simulink model "s_c_nbe_m1k_dbg2"  (R2016b)
(part 3 of 55)

  phase0/2(in_delta) -> Reinterpret3/1
  Reinterpret8/1 -> Concat22/1
  Reinterpret1/1 -> Concat22/2
  Reinterpret2/1 -> Concat22/3
  Reinterpret3/1 -> Concat22/4
  phase1/1(in_initial) -> Reinterpret5/1
  delta_delay1/1(in_delta) -> Reinterpret4/1
  phase1/2(in_delta) -> Reinterpret6/1
  Reinterpret4/1 -> Concat3/2
  Reinterpret5/1 -> Concat3/3
  Reinterpret6/1 -> Concat3/4
  Reinterpret7/1 -> Concat3/1
  delay0/1(in_initial) -> Reinterpret8/1
  delay1/1(in_initial) -> Reinterpret7/1
  tl_cd0_control0/3(in_load_time_msw) -> Concat6/1
  tl_cd0_control/1(in_load_time_lsw) -> Concat6/2
  Constant42/1 -> tl_cd0_control/1(sim_1)
  Constant40/1 -> tl_cd0_control0/3(sim_3)
  Constant41/1 -> tl_cd0_control0/2(sim_2)
  Constant43/1 -> Delay12/1
  Delay12/1 -> tl_cd0_control0/1(sim_1)
  Concat6/1 -> pipeline136/1(d)
  tl_cd0_control0/2(in_load_immediate) -> pipeline135/1(d)
  tl_cd0_control0/1(in_arm) -> pipeline134/1(d)
  tl_cd1_control0/3(in_load_time_msw) -> Concat8/1
  tl_cd1_control/1(in_load_time_lsw) -> Concat8/2
  Constant47/1 -> tl_cd1_control/1(sim_1)
  Constant45/1 -> tl_cd1_control0/3(sim_3)
  Constant46/1 -> tl_cd1_control0/2(sim_2)
  Constant48/1 -> Delay13/1
  Delay13/1 -> tl_cd1_control0/1(sim_1)
  Concat8/1 -> pipeline143/1(d)
  tl_cd1_control0/2(in_load_immediate) -> pipeline138/1(d)
  tl_cd1_control0/1(in_arm) -> pipeline137/1(d)
  Subsystem7/1(per_sec) -> reorder_status1/1(out_dv_per_sec)
  [upg_reo_time] -> Subsystem1/3(time)
  [upg_reo_recv] -> Subsystem1/4(recv)
  [upg_reo_dv] -> Subsystem7/1(dv), Subsystem1/2(dv)
  [cnt_rst] -> Subsystem1/1(rst)
  Subsystem1/7(time_change) -> [reo_time_change]
  Logical5/1 -> Subsystem1/7(overflow_err)
  [upg_of80_p1] -> Logical5/2
  [upg_of80_p0] -> Logical5/1
  Subsystem1/8(timestep_err) -> [up_timestep_error]
  [upg_reo_disc] -> Subsystem1/5(discard_err)
  [upg_reo_relock] -> Subsystem1/6(relock_err)
  Subsystem1/1(timestep_err_cnt) -> reorder_status/1(out_timestep_err_cnt)
  Subsystem1/2(recv_err_cnt) -> reorder_status/2(out_receive_err_cnt)
  Subsystem1/3(discard_err_cnt) -> reorder_status/3(out_discard_cnt)
  Subsystem1/4(relock_err_cnt) -> reorder_status/4(out_relock_err_cnt)
  Subsystem1/5(overflow_err_cnt) -> reorder_status/5(out_overflow_err_cnt)
  Subsystem1/6(dv_cnt) -> reorder_status/6(out_dv_cnt)
  forty_gbe/7(rx_valid) -> pipeline73/1(d)
  pipeline73/1(q) -> [forty_gbe_rx_valid]
  pipeline134/1(q) -> [tl_cd0_arm]
  pipeline135/1(q) -> [tl_cd0_load_immediate]
  pipeline136/1(q) -> [tl_cd0_load_time]
  pipeline138/1(q) -> [tl_cd1_load_immediate]
  pipeline137/1(q) -> [tl_cd1_arm]
  pipeline143/1(q) -> [tl_cd1_load_time]
  [gbe_txen] -> Logical4/2
  [force_gbe_txen] -> Logical6/2
  Logical6/1 -> Logical4/1
  [upg_sperr_magic] -> Subsystem33/2(in0)
  [upg_sperr_len] -> Subsystem33/5(in3)
  [upg_sperr_hdr] -> Subsystem33/3(in1)
  [upg_sperr_pad] -> Subsystem33/4(in2)
  Subsystem33/5(out4) -> unpack_status/5(out_time_err_cnt)
  [upg_sperr_time] -> Subsystem33/6(in4)
  Subsystem33/4(out3) -> unpack_status/4(out_pkt_len_err_cnt)
  Subsystem33/3(out2) -> unpack_status/3(out_pad_err_cnt)
  Subsystem33/2(out1) -> unpack_status/2(out_header_err_cnt)
  Subsystem33/1(out0) -> unpack_status/1(out_magic_err_cnt)
  [cnt_rst] -> Subsystem4/1(rst), Subsystem33/1(rst)
  Logical3/1 -> Subsystem4/2(in0)
  Subsystem4/1(out0) -> unpack_status1/1(out_pkt_cnt)
  [upg_sp_dv] -> Logical3/2
  [upg_sp_eof] -> Logical3/1
  unpack_and_reorder/5(spead_timestamp) -> [spead_timestamp]
  sync_gen/6(waiting) -> [sync_armed]
  [up_timestep_error] -> Logical15/1
  [sys_rst] -> Logical8/1
  Logical8/1 -> edge_detect17/1(in)
  [time_diff_error] -> Logical15/4
  [cd_error] -> Logical15/2
  [ct_error] -> Logical15/3
  edge_detect17/1(out) -> [sys_relock], Register/2
  [pack_sync] -> Register/3, Register/1
  unpack_and_reorder/4(recvd) -> ts_tvg/6(recvd_in)
  unpack_and_reorder/1(d160) -> ts_tvg/3(data_in)
  unpack_and_reorder/2(dv) -> ts_tvg/4(dv_in)
  unpack_and_reorder/3(time) -> ts_tvg/5(time_in)
  pipeline7/1(q) -> [unpack_d160]
  pipeline8/1(q) -> [unpack_dv]
  pipeline17/1(q) -> [unpack_timestamp]
  ts_tvg/1(d160) -> pipeline7/1(d)
  ts_tvg/2(dv) -> pipeline8/1(d)
  ts_tvg/3(time) -> pipeline17/1(d)
  ts_tvg/4(recvd) -> Terminator14/1
  [ts_tvg_en] -> ts_tvg/1(tvg_en)
  [pipeline_stall] -> ts_tvg/2(stall_pipeline)
  edge_detect4/1(out) -> pipeline63/1(d)
  control/7(in_cnt_rst) -> edge_detect1/1(in)
  edge_detect1/1(out) -> pipeline15/1(d)
  control/3(in_gbe_rst) -> pipeline70/1(d)
  control/1(in_sys_rst) -> pipeline39/1(d)
  pipeline39/1(q) -> [sys_rst]
  pipeline63/1(q) -> [clr_status]
  pipeline70/1(q) -> [gbe_rst]
  pipeline78/1(q) -> [gbe_txen]
  pipeline14/1(q) -> [tvg_adc0_en]
  pipeline15/1(q) -> [cnt_rst]
  control/5(in_tvg_adc0) -> pipeline14/1(d)
  edge_detect3/1(out) -> pipeline57/1(d)
  pipeline57/1(q) -> [gbe_cnt_rst]
  control/8(in_gbe_cnt_rst) -> edge_detect3/1(in)
  control/4(in_gbe_txen) -> pipeline78/1(d)
  control/2(in_status_clr) -> edge_detect4/1(in)
  pipeline60/1(q) -> [adc_snap_arm]
  control/9(in_adc_snap_arm) -> pipeline60/1(d)
  control/10(in_adc_snap_trig_select) -> pipeline58/1(d)
  pipeline58/1(q) -> [adc_snap_trig_source]
  pipeline69/1(q) -> [ct_tvg_en]
  control/11(in_ct_tvg_en) -> pipeline69/1(d)
  pipeline65/1(q) -> [up_dbg_rst]
  control/12(in_unpack_debug_reset) -> pipeline65/1(d)
  control/13(in_cd_bypass) -> pipeline131/1(d)
  pipeline131/1(q) -> Convert2/1
  pipeline107/1(q) -> [tvg_adc1_en]
  control/6(in_tvg_adc1) -> pipeline107/1(d)
  control/14(in_gbe_stopmux) -> pipeline98/1(d)
  pipeline98/1(q) -> [gbe_stopmux]
  control/15(in_pfb_bypass) -> pipeline74/1(d)
  pipeline74/1(q) -> [pfb_bypass]
  control/16(in_ts_tvg_en) -> pipeline148/1(d)
  pipeline148/1(q) -> [ts_tvg_en]
  control/17(in_force_gbe_txen) -> pipeline30/1(d)
  pipeline30/1(q) -> [force_gbe_txen]
  control/18(in_snap_stop_mux_sel) -> pipeline127/1(d)
  control/19(in_snap_reord_mux_we_sel) -> pipeline128/1(d)
  pipeline127/1(q) -> [snap_stop_mux_sel]
  pipeline128/1(q) -> [snap_reord_mux_we_sel]
  control/20(in_local_time_source) -> pipeline6/1(d)
  edge_detect6/1(out) -> pipeline164/1(d)
  pipeline164/1(q) -> [local_time_capture]
  pipeline6/1(q) -> [local_time_src]
  control/21(in_local_time_capture) -> edge_detect6/1(in)
  control/22(in_time_diff_check_en) -> pipeline62/1(d)
  pipeline62/1(q) -> [time_diff_check_en]
  control/23(in_auto_rst_enable) -> pipeline132/1(d)
  pipeline132/1(q) -> [auto_rst_enable]
  pipeline18/1(q) -> [pipeline_stall]
  control/24(in_pipeline_stall) -> pipeline18/1(d)
  Counter12/1 -> Slice13/1
  Slice13/1 -> edge_detect8/1(in)
  Logical15/1 -> Logical11/2, Counter12/1
  Logical11/1 -> [fault_detected]
  Register6/1 -> Inverter6/1
  Register/1 -> [synced], posedge_delay/1(In1)
  posedge_delay/1(Out1) -> [synced_delay]
  [board_in_fault] -> Inverter1/1
  Inverter1/1 -> Logical6/1
  [synced] -> Inverter2/1
  Inverter2/1 -> Counter1/2
  [pack_sync] -> Counter1/1
  Counter1/1 -> Slice16/1
  Slice16/1 -> edge_detect5/1(in)
  edge_detect8/1(out) -> Logical11/1
  [sys_relock] -> Delay57/1
  Inverter6/1 -> [board_in_fault]
  Delay57/1 -> Register6/2
  [synced_delay] -> edge_detect9/1(in)
  edge_detect9/1(out) -> Register6/3, Register6/1
  edge_detect5/1(out) -> [sync_timeout]
  [auto_rst_enable] -> Logical7/1
  [synced_delay] -> Logical7/2
  [fault_detected] -> Logical7/3
  [sync_timeout] -> Logical14/2
  [auto_rst_enable] -> Logical14/1
  Logical14/1 -> Logical8/2
  Logical7/1 -> Logical8/3
  Counter2/1 -> pipeline29/1(d)
  Constant26/1 -> eq1/2(data_in)
  Constant4/1 -> eq1/3(we)
  eq1/1(data_out) -> Terminator3/1
  Counter4/1 -> pipeline27/1(d)
  Constant24/1 -> eq0/2(data_in)
  Constant25/1 -> eq0/3(we)
  eq0/1(data_out) -> Terminator4/1
  Delay51/1 -> [q_sync]
  Delay52/1 -> [q_dv]
  Delay53/1 -> Terminator19/1
  Delay50/1 -> Terminator21/1
  pipeline27/1(q) -> eq0/1(addr)
  pipeline29/1(q) -> eq1/1(addr)
  [fdfs_sync] -> Delay51/1, pipeline42/1(d)
  [fdfs_dv] -> Delay52/1, pipeline41/1(d)
  pipeline41/1(q) -> Counter4/2
  pipeline42/1(q) -> Counter4/1
  pipeline45/1(q) -> Counter2/2
  [fdfs_sync] -> Delay53/1, pipeline25/1(d)
  [fdfs_dv] -> Delay50/1, pipeline45/1(d)
  pipeline25/1(q) -> Counter2/1
  pipeline23/1(q) -> [outfreq_stopmux]
  ct_debug/6(in_outfreq_stopmux) -> pipeline23/1(d)
  pipeline24/1(q) -> [out_stopmux]
  ct_debug/5(in_out_stopmux) -> pipeline24/1(d)
  pipeline55/1(q) -> [wrrd_stopmux]
  ct_debug/3(in_wrrd_stopmux) -> pipeline55/1(d)
  pipeline56/1(q) -> [in_stopmux]
  ct_debug/1(in_in_stopmux) -> pipeline56/1(d)
  pipeline122/1(q) -> [ct_snap_arm]
  pipeline22/1(q) -> edge_detect7/1
  ct_debug/8(in_snap_trig) -> pipeline22/1(d)
  ct_debug/7(in_snap_arm) -> pipeline122/1(d)
  edge_detect7/1 -> [ct_snap_trig]
  ct_debug/2(in_in_trigmux) -> pipeline150/1(d)
  pipeline150/1(q) -> [in_trigmux]
  ct_debug/4(in_obuf_stopmux) -> pipeline167/1(d)
  pipeline167/1(q) -> [obuf_stopmux]
  ct_debug/9(in_snap_wesel) -> pipeline81/1(d)
  pipeline81/1(q) -> [ct_snap_wesel]
  pipeline157/1(q) -> [ct_snap_trigsel]
  ct_debug/10(in_snap_trigsel) -> pipeline157/1(d)
  pipeline166/1(q) -> [ct_snap_circsel]
  ct_debug/11(in_snap_circsel) -> pipeline166/1(d)
  bus_create2/1(bus_out) -> [tvgtone_level0]
  bus_create3/1(bus_out) -> [tvgtone_level1]
  tvg_tone_levels/2(in_p0i) -> bus_create2/2(in2)
  tvg_tone_levels/3(in_p1r) -> bus_create3/1(in1)
  tvg_tone_levels/4(in_p1i) -> bus_create3/2(in2)
  tvg_tone_levels/1(in_p0r) -> bus_create2/1(in1)
  tvg_tone_targets/1(in_p0) -> Slice18/1
  tvg_tone_targets/2(in_p1) -> Slice19/1
  Constant51/1 -> tvg_tone_targets/1(sim_1)
  Constant52/1 -> tvg_tone_targets/2(sim_2)
  Constant37/1 -> tvg_tone_levels/4(sim_4)
  Constant8/1 -> tvg_tone_levels/1(sim_1)
  Constant27/1 -> tvg_tone_levels/3(sim_3)
  Constant9/1 -> tvg_tone_levels/2(sim_2)
  we_delay49/1(q) -> [ct_tag_insert_sel]
  edge_detect2/1 -> [ct_rst_err_latch]
  we_delay47/1(q) -> edge_detect2/1
  we_delay48/1(q) -> [ct_fake_data_error]
  we_delay13/1(q) -> [ct_tvg_en]
  we_delay50/1(q) -> [ct_tvg_en2]
  Constant12/1 -> ct_control0/5(sim_5)
  Constant21/1 -> ct_control0/4(sim_4)
  Constant20/1 -> ct_control0/3(sim_3)
  Constant22/1 -> ct_control0/2(sim_2)
  Constant15/1 -> ct_control0/1(sim_1)
  ct_control0/1(in_tvg_en) -> we_delay13/1(d)
  ct_control0/2(in_tvg_en2) -> we_delay50/1(d)
  ct_control0/3(in_rst_err_latch) -> we_delay47/1(d)
  ct_control0/4(in_fake_error) -> we_delay48/1(d)
  ct_control0/5(in_tag_insert) -> we_delay49/1(d)
  we_delay126/1(q) -> [obuf_read_gap]
  ct_control0/6(in_obuf_read_gap) -> we_delay126/1(d)
  Constant30/1 -> ct_control0/6(sim_6)
  we_delay41/1(q) -> [ct_num_xeng]
  we_delay112/1(q) -> [ct_num_xeng_recip]  "NUM_X_RECIP"
  ct_control1/2(in_num_x_recip) -> we_delay112/1(d)
  ct_control1/1(in_num_x) -> we_delay41/1(d)
  we_delay114/1(q) -> [ct_x_per_board]
  ct_control1/3(in_x_per_board) -> we_delay114/1(d)
  we_delay113/1(q) -> [ct_chans_per_board]
  ct_control2/1(in_chans_per_x) -> we_delay39/1(d)
  ct_control2/2(in_chans_per_board) -> we_delay113/1(d)
  we_delay115/1(q) -> [ct_x_per_board_recip]
  ct_control1/4(in_x_per_board_recip) -> we_delay115/1(d)
  we_delay38/1(q) -> [ct_num_x_boards]
  ct_control3/1(in_num_x_boards) -> we_delay38/1(d)
  we_delay37/1(q) -> [ct_num_x_boards_recip]
  ct_control3/2(in_num_x_boards_recip) -> we_delay37/1(d)
  ct_control3/3(in_chans_per_x_recip) -> we_delay124/1(d)
  Constant49/1 -> ct_control1/1(sim_1)
  Constant53/1 -> ct_control1/2(sim_2)
  Constant33/1 -> ct_control1/3(sim_3)
  Constant23/1 -> ct_control2/1(sim_1)
  Constant50/1 -> ct_control2/2(sim_2)
  Constant54/1 -> ct_control1/4(sim_4)
  Constant32/1 -> ct_control3/1(sim_1)
  Constant14/1 -> ct_control3/2(sim_2)
  Constant44/1 -> ct_control3/3(sim_3)
  Slice18/1 -> [tvgtone_p0]
  Slice19/1 -> [tvgtone_p1]
  Slice36/1 -> we_delay116/1(d)
  Constant38/1 -> ct_control4/1(sim_1)
  ct_control4/1(in_ct_board_offset) -> Slice36/1
  ct_control5/1(in_ct_freq_gen_offset) -> we_delay117/1(d)
  Constant39/1 -> ct_control5/1(sim_1)
  we_delay116/1(q) -> [ct_board_hmc_offset]
  we_delay117/1(q) -> [ct_freq_gen_offset]
  we_delay124/1(q) -> [ct_chans_per_x_recip]
  we_delay39/1(q) -> [ct_chans_per_x]  "PER_X"
  pipeline196/1(q) -> ddc_dvalid_cnt/1(out_reg)
  pipeline197/1(q) -> ddc_sync_cnt/1(out_reg)
  pipeline198/1(q) -> DDC/8(scale1)
  pipeline199/1(q) -> DDC/5(scale0)
  pipeline207/1(q) -> [cwg_tp]
  cwg2/1(bus_out) -> pipeline207/1(d)
  cwg2/3(rpt_rst) -> Terminator17/1
  cwg2/2(dvalid) -> Terminator15/1
  Constant55/1 -> freq_cwg_tp/1(sim_1)
  Constant56/1 -> scale_cwg_tp/1(sim_1)
  freq_cwg_tp/1(in_frequency) -> pipeline209/1(d)
  scale_cwg_tp/1(in_scale) -> pipeline40/1(d)
  pipeline208/1(q) -> cwg2/3(rst)
  rpt_en_cwg_tp/1(in_en) -> pipeline210/1(d)
  rpt_length_cwg_tp/1(in_repeat_length) -> pipeline44/1(d)
  Constant58/1 -> cwg2/6(en)
  [sys_rst] -> pipeline208/1(d)
  Constant59/1 -> rpt_en_cwg_tp/1(sim_1)
  Constant60/1 -> rpt_length_cwg_tp/1(sim_1)
  pipeline40/1(q) -> cwg2/2(scale)
  pipeline209/1(q) -> cwg2/1(freq)
  pipeline210/1(q) -> cwg2/4(repeat_en)
  pipeline44/1(q) -> cwg2/5(repeat_length)
  edge_detect14/1(out) -> Delay32/1
  pipeline126/1(q) -> snap_ddc_out/4(we)
  pipeline86/1(q) -> snap_ddc_out/1(in_ddc0)
  pipeline161/1(q) -> snap_ddc_out/2(in_dv)
  pipeline82/1(q) -> snap_ddc_out/3(in_sync)
  trig_time_msw/1(in_msw) -> pipeline213/1(d)
  trig_time_lsw/1(in_lsw) -> pipeline214/1(d)
  Concat13/1 -> Relational10/1
  pipeline213/1(q) -> Concat13/1
  pipeline214/1(q) -> Concat13/2
  [time80_48] -> Relational10/2
  pipeline215/1(q) -> bus_expand18/1(bus_in)
  [valid80] -> Slice5/1
  Slice14/1 -> pipeline211/1(d)
  [time80_48] -> Slice14/1
  pipeline211/1(q) -> snap_adc0/13(extra_timestamp)
  [d80_adc0] -> pipeline215/1(d)
  bus_expand18/4(out5) -> snap_adc0/4(in_p0_d3)
  bus_expand18/5(out4) -> snap_adc0/5(in_p0_d4)
  bus_expand18/1(msb_out8) -> snap_adc0/1(in_p0_d0)
  bus_expand18/2(out7) -> snap_adc0/2(in_p0_d1)
  bus_expand18/3(out6) -> snap_adc0/3(in_p0_d2)
  bus_expand18/6(out3) -> snap_adc0/6(in_p0_d5)
  bus_expand18/7(out2) -> snap_adc0/7(in_p0_d6)
  bus_expand18/8(lsb_out1) -> snap_adc0/8(in_p0_d7)
  pipeline202/1(q) -> snap_adc0/11(we)
  Relational10/1 -> Logical12/1
  [valid80] -> pipeline162/1(d)
  Logical12/1 -> snap_adc0/12(trig)
  pipeline162/1(q) -> Logical12/2
  [delay_d1] -> [pfbin_d1]
  Convert2/1 -> [cd_bypass]
  Constant61/1 -> int_cwg_en/1(sim_1)
  [cwg_tp] -> Terminator2/1
  int_cwg_en/1(in_int_cwg) -> Delay33/1, edge_detect14/1(in), Terminator10/1, Terminator11/1, Terminator6/1
  Delay32/1 -> Terminator8/1
  Delay33/1 -> Terminator5/1
  [pfbin_sync] -> [ddc_sync_in]
  [pfbin_dv] -> [ddc_dv_in]
  [ddc_dv_in] -> DDC/2(dvalid)
  [ddc_sync_in] -> DDC/1(sync)
  [pfbin_d0] -> [ddc_pol0_in]
  bus_expand7/4(out5) -> pipeline224/1(d)
  bus_expand7/5(out4) -> pipeline223/1(d)
  bus_expand7/2(out7) -> pipeline226/1(d)
  bus_expand7/3(out6) -> pipeline225/1(d)
  bus_expand7/6(out3) -> pipeline222/1(d)
  bus_expand7/7(out2) -> pipeline221/1(d)
  bus_expand7/8(lsb_out1) -> pipeline220/1(d)
  bus_expand7/1(msb_out8) -> pipeline227/1(d)
  pipeline61/1(q) -> snap_ddc_in/11(we)
  pipeline218/1(q) -> snap_ddc_in/10(in_dv)
  pipeline219/1(q) -> snap_ddc_in/9(in_sync)
  pipeline220/1(q) -> snap_ddc_in/8(in_p0_d7)
  pipeline221/1(q) -> snap_ddc_in/7(in_p0_d6)
  pipeline222/1(q) -> snap_ddc_in/6(in_p0_d5)
  pipeline223/1(q) -> snap_ddc_in/5(in_p0_d4)
  pipeline224/1(q) -> snap_ddc_in/4(in_p0_d3)
  pipeline225/1(q) -> snap_ddc_in/3(in_p0_d2)
  pipeline226/1(q) -> snap_ddc_in/2(in_p0_d1)
  pipeline227/1(q) -> snap_ddc_in/1(in_p0_d0)
  pipeline68/1(q) -> snap_adc0/10(in_dv)
  pipeline83/1(q) -> snap_adc0/9(in_sync)
  Slice5/1 -> pipeline68/1(d), pipeline202/1(d)
  [sync80] -> pipeline83/1(d)
  [ddc_pol0_in] -> bus_expand7/1(bus_in)
  [ddc_sync_in] -> pipeline219/1(d), snap_ddc_in/12(trig)
  [ddc_dv_in] -> pipeline218/1(d), pipeline61/1(d)
  pipeline231/1(q) -> bus_expand10/1(bus_in)
  bus_expand10/4(out5) -> snap_mix/4(in_p0_d3)
  bus_expand10/5(out4) -> snap_mix/5(in_p0_d4)
  bus_expand10/1(msb_out8) -> snap_mix/1(in_p0_d0)
  bus_expand10/2(out7) -> snap_mix/2(in_p0_d1)
  bus_expand10/3(out6) -> snap_mix/3(in_p0_d2)
  bus_expand10/6(out3) -> snap_mix/6(in_p0_d5)
  bus_expand10/7(out2) -> snap_mix/7(in_p0_d6)
  bus_expand10/8(lsb_out1) -> snap_mix/8(in_p0_d7)
  pipeline141/1(q) -> snap_mix/11(we)
  pipeline232/1(q) -> snap_mix/10(in_dv)
  pipeline242/1(q) -> snap_mix/9(in_sync)
  [mix_80_0] -> pipeline231/1(d)
  [mix_dvalid] -> pipeline141/1(d), pipeline232/1(d)
  [mix_sync] -> pipeline242/1(d), snap_mix/12(trig)
  [ddc_sync] -> pipeline82/1(d), snap_ddc_out/5(trig)
  [ddc_pol0] -> pipeline86/1(d)
  [ddc_dvalid] -> pipeline126/1(d), pipeline161/1(d)
  [pfbin_d1] -> DDC/6(pol1_data)
  [ddc_pol0_in] -> DDC/3(pol0_data)
  [sync80] -> [delay_sync]
  [d80_adc0] -> [delay_d1], [delay_d0]
  [valid80] -> [delay_dv]
  pipeline11/1(q) -> bus_expand1/1(bus_in)
  [unpack_dv] -> Slice9/1, Slice3/1, snap_unpack/12(trig)
  Slice1/1 -> pipeline10/1(d)
  [unpack_timestamp] -> Slice1/1
  pipeline10/1(q) -> snap_unpack/13(extra_timestamp)
  bus_expand3/1(msb_out2) -> pipeline11/1(d)
  bus_expand1/4(out5) -> snap_unpack/4(in_p0_d3)
  bus_expand1/5(out4) -> snap_unpack/5(in_p0_d4)
  bus_expand1/1(msb_out8) -> snap_unpack/1(in_p0_d0)
  bus_expand1/2(out7) -> snap_unpack/2(in_p0_d1)
  bus_expand1/3(out6) -> snap_unpack/3(in_p0_d2)
  bus_expand1/6(out3) -> snap_unpack/6(in_p0_d5)
  bus_expand1/7(out2) -> snap_unpack/7(in_p0_d6)
  bus_expand1/8(lsb_out1) -> snap_unpack/8(in_p0_d7)
  pipeline5/1(q) -> snap_unpack/11(we)
  pipeline26/1(q) -> snap_unpack/10(in_dv)
  pipeline32/1(q) -> snap_unpack/9(in_sync)
  Slice3/1 -> pipeline5/1(d), pipeline26/1(d)
  [sync80] -> pipeline32/1(d)
  [unpack_d160] -> bus_expand3/1(bus_in)
  pipeline33/1(q) -> bus_expand4/1(bus_in)
  bus_expand4/1(msb_out8) -> snap_unpack1/1(in_p0_d0)
  bus_expand4/2(out7) -> snap_unpack1/2(in_p0_d1)
  bus_expand4/4(out5) -> snap_unpack1/4(in_p0_d3)
  bus_expand4/3(out6) -> snap_unpack1/3(in_p0_d2)
  bus_expand4/5(out4) -> snap_unpack1/5(in_p0_d4)
  bus_expand4/6(out3) -> snap_unpack1/6(in_p0_d5)
  bus_expand4/7(out2) -> snap_unpack1/7(in_p0_d6)
  bus_expand4/8(lsb_out1) -> snap_unpack1/8(in_p0_d7)
  bus_expand3/2(lsb_out1) -> pipeline33/1(d)
  Slice9/1 -> snap_unpack1/12(trig), pipeline34/1(d), pipeline35/1(d)
  pipeline34/1(q) -> snap_unpack1/10(in_dv)
  pipeline35/1(q) -> snap_unpack1/11(we)
  pipeline36/1(q) -> snap_unpack1/9(in_sync)
  [sync80] -> pipeline36/1(d)
  pipeline37/1(q) -> snap_unpack1/13(extra_timestamp)
  [unpack_timestamp] -> Slice10/1
  Slice10/1 -> pipeline37/1(d)
  Constant5/1 -> [cd_error], [ct_error]
  Slice17/1 -> local_time_lsw/1(out_timestamp_lsw)
  Slice15/1 -> Convert1/1
  [local_time_capture] -> Delay31/1
  pipeline19/1(q) -> Slice17/1, Slice15/1
  [local_time_src] -> Mux/1
  [time80_48] -> Delay14/1
  [valid80] -> Delay14/2
  Delay14/1 -> Register1/1, AddSub/2
  [pfb_time] -> Delay10/1
  [pfb_dv] -> Delay10/2
  Delay11/1 -> Register3/1, AddSub/1
  [flag_dvalid] -> Delay11/2
  [pack_sync_time] -> Delay11/1
  Convert1/1 -> local_time_msw/1(out_timestamp_msw)
  AddSub/1 -> time_difference/1(out_time_difference), Relational4/1
  Relational4/1 -> Logical/1
  Logical/1 -> [time_diff_error]
  time_check/1(in_max_difference) -> Relational4/2
  [time_diff_check_en] -> Logical/2
  Delay31/1 -> Register3/2, Register2/2, Register4/2, Register1/2
  Delay10/1 -> Register2/1
  [spead_timestamp] -> Register4/1
  Register4/1 -> Mux/2
  Register1/1 -> Mux/3
  Register2/1 -> Mux/4
  Register3/1 -> Mux/5
  Mux/1 -> pipeline19/1(d)
  [cnt_rst] -> Subsystem2/1(rst)
  [synced] -> Delay38/1
  [sync_armed] -> Delay39/1
  [board_in_fault] -> Delay48/1
  [q_sync] -> Subsystem19/5(in3)
  [pfb_sync] -> Subsystem19/3(in1)
  [fdfs_sync] -> Subsystem19/4(in2)
  [sync80] -> Subsystem19/2(in0)
  [cnt_rst] -> Subsystem19/1(rst)
  Subsystem19/2(out1) -> sync_status2/2(out_sync_pfb_cnt)
  Subsystem19/1(out0) -> sync_status2/1(out_sync80_cnt)
  Subsystem19/3(out2) -> sync_status2/3(out_sync_fdfs_cnt)
  [pack_sync] -> Subsystem12/4(in2)
  [flag_sync] -> Subsystem12/3(in1)
  [ct_sync] -> Subsystem12/2(in0)
  [cnt_rst] -> Subsystem12/1(rst)
  [synced_delay] -> Subsystem2/2(armed)
  [sync_timeout] -> Subsystem2/3(in1)
  [time_diff_error] -> Subsystem2/4(in2)
  [up_timestep_error] -> Subsystem2/5(in3)
  [cd_error] -> Subsystem2/6(in4)
  [ct_error] -> Subsystem2/7(in5)
  Delay48/1 -> sync_status0/2(out_board_in_fault)
  Delay38/1 -> sync_status0/3(out_synced)
  Delay39/1 -> sync_status0/4(out_sync_armed)
  Subsystem12/1(out0) -> sync_status0/5(out_sync_ct)
  Subsystem12/2(out1) -> sync_status0/6(out_sync_flag)
  Subsystem12/3(out2) -> sync_status0/7(out_sync_pack)
  Subsystem2/1(Out1) -> sync_status1/1(out_timeout_resync_cnt)
  Subsystem2/2(Out2) -> sync_status1/2(out_time_diff_resync_cnt)
  Subsystem2/3(Out3) -> sync_status1/3(out_timestep_resync_cnt)
  [synced_delay] -> Delay58/1
  Delay58/1 -> sync_status0/1(out_synced_delay)
  Subsystem19/4(out3) -> sync_status2/4(out_sync_quant_cnt)
  Subsystem2/4(Out4) -> sync_status1/4(out_cd_resync_cnt)
  Subsystem2/5(Out5) -> sync_status1/5(out_ct_resync_cnt)
  [hmc_dvalid] -> Subsystem26/1(In1)
  Subsystem26/1(Out1) -> pipeline200/1(d)
  [dvalid_tl_cd0] -> Subsystem25/1(In1)
  Subsystem25/1(Out1) -> pipeline201/1(d)
  pipeline200/1(q) -> cd_out_dv_rate/1(out_reg)
  pipeline201/1(q) -> cd_in_dv_rate/1(out_reg)
  [valid80] -> [dvalid_tl_cd0], [hmc_dvalid]
  [ct_dv] -> Subsystem8/1(In1)
  Subsystem8/1(Out1) -> pipeline165/1(d)
  [ct_pktstart] -> we_delay1/1(d)
  [ct_dv] -> we_delay2/1(d)
  we_delay1/1(q) -> pktlen_check/1(pkt_start)
  we_delay2/1(q) -> dv_block_check/1(dv), pktlen_check/2(dv)
  pktlen_check/1(error) -> we_delay7/1(d)
  dv_block_check/1(error) -> we_delay29/1(d)
  [cnt_rst] -> Subsystem6/1(rst)
  we_delay7/1(q) -> [ct_pktlen_err], Subsystem6/2(in0)
  we_delay29/1(q) -> [ct_dvblk_err], Subsystem6/3(in1)
  Subsystem6/1(out0) -> pipeline169/1(d)
  Subsystem6/2(out1) -> pipeline168/1(d)
  [q_dv] -> Subsystem17/1(In1)
  Subsystem17/1(Out1) -> pipeline163/1(d)
  [cnt_rst] -> Subsystem10/1(rst)
  [q_sync] -> Subsystem10/2(in0)
  Constant13/1 -> Subsystem10/3(in1)
  Constant31/1 -> Subsystem10/4(in2)
  [ct_sync] -> Subsystem10/5(in3)
  Subsystem10/1(out0) -> pipeline160/1(d)
  Subsystem10/2(out1) -> pipeline159/1(d)
  Subsystem10/3(out2) -> pipeline158/1(d)
  Subsystem10/4(out3) -> pipeline155/1(d)
  pipeline155/1(q) -> ct_sync_cnt/4(out_sync_out)
  pipeline158/1(q) -> ct_sync_cnt/3(out_rd_sync_cnt)
  pipeline159/1(q) -> ct_sync_cnt/2(out_rd_addr_arm_cnt)
  pipeline160/1(q) -> ct_sync_cnt/1(out_sync_in)
  pipeline163/1(q) -> ct_in_dv_rate/1(out_reg)
  pipeline165/1(q) -> ct_out_dv_rate/1(out_reg)
  pipeline168/1(q) -> ct_dv_err/2(out_dvblock_err_cnt)
  pipeline169/1(q) -> ct_dv_err/1(out_pktlen_err_cnt)
  [q_sync] -> [ct_pktstart]
  [q_dv] -> [ct_dv]
  [clr_status] -> Subsystem3/1(rst)
  Slice6/1 -> Subsystem3/2(in0)
  [pfb_of] -> Slice6/1, Slice20/1
  Slice20/1 -> Subsystem3/3(in1)
  [pfb_sync] -> Subsystem3/4(in2)
  Subsystem3/3(out2) -> pipeline193/1(d)
  Subsystem3/1(out0) -> pipeline195/1(d)
  Subsystem3/2(out1) -> pipeline194/1(d)
  Constant17/1 -> [pfb_of]
  Counter7/1 -> pipeline191/1(d)
  [pfb_sync] -> Counter7/2
  [cnt_rst] -> Counter7/1
  [pfb_dv] -> Counter8/2
  [cnt_rst] -> Counter8/1
  Counter8/1 -> pipeline192/1(d)
  pipeline191/1(q) -> nb_sync_cnt/1(out_reg)
  pipeline192/1(q) -> nb_dvalid_cnt/1(out_reg)
  pipeline193/1(q) -> pfb_status/3(out_sync_cnt)
  pipeline194/1(q) -> pfb_status/2(out_pol1_or_err_cnt)
  pipeline195/1(q) -> pfb_status/1(out_pol0_or_err_cnt)
  Constant28/1 -> [ct_sync]
  Delay72/1 -> [flag_sync]
  Delay75/1 -> [flag_misc]
  Delay73/1 -> [flag_dvalid]
  Delay74/1 -> [flag_time]
  Delay43/1 -> time_gen1/4(rd_sync_in)
  Delay59/1 -> time_gen1/6(rd_misc_in)
  Delay/1 -> Delay43/1  "gapsync"
  Delay3/1 -> Delay47/1  "gapdata"
  Mux1/1 -> Delay59/1  "gapvalid"
  [time80] -> Slice2/1
  Delay47/1 -> time_gen1/5(rd_en)
  time_gen1/1(rd_sync_out) -> Delay72/1
  time_gen1/4(rd_misc_out) -> Delay75/1
  time_gen1/2(rd_dvalid) -> Delay73/1
  time_gen1/3(rd_val_out) -> Delay74/1
  Slice2/1 -> time_gen1/3(wr_val_in)
  [ct_tvg_en2] -> Mux1/1
  Delay17/1 -> Mux1/2
  Delay18/1 -> tvg/1(sync), Delay/1
  Delay16/1 -> tvg/2(dv), Delay3/1
  tvg/1(data256) -> Mux1/3
  [flag_dvalid] -> Subsystem13/1(In1)
  Subsystem13/1(Out1) -> pipeline186/1(d)
  [s256_v] -> Subsystem11/1(In1)
  Subsystem11/1(Out1) -> pipeline187/1(d)
  pipeline38/1(q) -> Convert3/1
  pipeline46/1(q) -> [ip_per_x]
  pipeline47/1(q) -> [num_x]
  x_setup/1(in_f_per_x) -> pipeline38/1(d)
  x_setup/2(in_ip_per_x) -> pipeline46/1(d)
  x_setup/3(in_num_x) -> pipeline47/1(d)
  pipeline52/1(q) -> [pack_snap_arm]
  x_setup/4(in_snap_arm) -> pipeline52/1(d)
  pipeline48/1(q) -> [pktstart_sel]
  x_setup/5(in_pktstart_mux) -> pipeline48/1(d)
  [s256_v] -> pack_block_check/1(dv)
  [cnt_rst] -> Subsystem14/1(rst)
  Subsystem14/1(out0) -> pipeline188/1(d)
  pack_block_check/1(error) -> [pack_dv_err], Subsystem14/2(in0)
  pipeline49/1(q) -> [pack_mux]
  x_setup/6(in_pack_mux) -> pipeline49/1(d)
  Convert3/1 -> [f_per_x]
  [ct_d256] -> Delay17/1
  [ct_dv] -> Delay16/1
  [ct_sync] -> Delay18/1
  x_setup/7(in_pktoffset_sel) -> pipeline54/1(d)
  pipeline54/1(q) -> [pktoffset_sel]
  iptx_base/1(in_reg) -> pipeline53/1(d)
  pipeline53/1(q) -> [tx_ip_base]
  tx_metadata/1(in_porttx) -> pipeline50/1(d)
  tx_metadata/2(in_board_id) -> pipeline51/1(d)
  pipeline50/1(q) -> [tx_port]
  pipeline51/1(q) -> [tx_board_id]
  Delay64/1 -> Delay68/1
  Delay4/1 -> Delay5/1
  Delay5/1 -> Delay60/1
  Delay60/1 -> Delay64/1
  Delay68/1 -> [flag_pktstart]
  Delay1/1 -> Delay6/1
  Delay6/1 -> Delay61/1
  Delay65/1 -> Delay69/1
  Delay69/1 -> [flag_pktfreq]
  Delay61/1 -> Delay65/1
  Delay15/1 -> Delay7/1
  Delay7/1 -> Delay62/1
  Delay62/1 -> Delay66/1
  Delay66/1 -> Delay70/1
  Delay70/1 -> [flag_pktxindex]
  Delay19/1 -> Delay20/1
  Delay20/1 -> Delay63/1
  Delay63/1 -> Delay67/1
  Delay67/1 -> Delay71/1
  Delay71/1 -> [flag_pktxoffset]
  [ct_pkt_x_index] -> Delay15/1
  [ct_pkt_x_offset] -> Delay19/1
  [ct_pktfreq] -> Delay1/1
  [ct_pktstart] -> Delay4/1
  [flag_sync] -> packetiser/1(sync_in)
  [flag_dvalid] -> packetiser/2(en)
  [flag_pktstart] -> packetiser/5(pkt_start)
  [flag_pktxoffset] -> packetiser/7(pkt_x_offset)
  [tx_ip_base] -> packetiser/9(base_ip)
  [tx_port] -> packetiser/10(base_port)
  Constant3/1 -> concat1/2
  [flag_time] -> concat1/1
  [flag_misc] -> packetiser/3(din)
  concat1/1 -> [pack_sync_time], packetiser/4(timestamp)
  Delay82/1 -> [s256_d]
  Delay83/1 -> [s256_v]
  Delay84/1 -> [s256_eof]
  Delay85/1 -> [s256_of]
  Delay86/1 -> [s256_ip]
  Delay87/1 -> [s256_port]
  Delay88/1 -> [pack_sync]
  packetiser/1(dout) -> Delay82/1
  packetiser/2(dvalid) -> Delay83/1
  packetiser/3(eof) -> Delay84/1
  packetiser/4(overflow) -> Delay85/1
  packetiser/5(destination_ip) -> Delay86/1
  packetiser/6(destination_port) -> Delay87/1
  packetiser/7(sync) -> Delay88/1
  [flag_pktfreq] -> Delay77/1
  Delay89/1 -> [s256_pktfreq]
  Delay77/1 -> Delay89/1
  [flag_pktxindex] -> Delay78/1
  Delay78/1 -> Delay90/1
  Delay90/1 -> [s256_pktxindex]
  [flag_pktxoffset] -> Delay79/1
  Delay79/1 -> Delay91/1
  Delay91/1 -> [s256_pktxoffset]
  [tx_board_id] -> packetiser/8(board_id)
  [flag_pktstart] -> Delay80/1
  Delay80/1 -> Delay92/1
  Delay92/1 -> [s256_pktstart]
  [sync80] -> time_gen1/1(wr_sync_in)
  [valid80] -> time_gen1/2(wr_en)
  [time80_48] -> Subsystem/1(time)
  [sync80] -> Subsystem/2(sync)
  [valid80] -> Subsystem/3(dv)
  Subsystem/1(msw) -> pipeline184/1(d)
  Subsystem/2(ls32) -> pipeline185/1(d)
  [flag_pktxindex] -> packetiser/6(pkt_x_index)
  [flag_time] -> Delay81/1
  Delay81/1 -> Delay93/1
  Delay93/1 -> [s256_time]
  time_gen1/5(epoch) -> Delay76/1
  Slice4/1 -> pipeline182/1(d)
  Slice11/1 -> pipeline183/1(d)
  Delay76/1 -> Concat10/1
  Constant16/1 -> Concat10/2
  Concat10/1 -> Slice4/1, Slice11/1, [flag_epoch]
  [flag_pktfreq] -> Subsystem27/3(value)
  [cnt_rst] -> Subsystem27/1(rst)
  [flag_dvalid] -> Subsystem27/2(en)
  Subsystem27/1(current) -> pipeline170/1(d)
  Subsystem27/3(min) -> pipeline172/1(d)
  Subsystem27/2(max) -> pipeline171/1(d)
  [flag_pktxindex] -> Subsystem28/3(value)
  [cnt_rst] -> Subsystem28/1(rst)
  [flag_dvalid] -> Subsystem28/2(en)
  Subsystem28/1(current) -> pipeline173/1(d)
  Subsystem28/3(min) -> pipeline175/1(d)
  Subsystem28/2(max) -> pipeline174/1(d)
  [flag_pktxoffset] -> Subsystem29/3(value)
  [cnt_rst] -> Subsystem29/1(rst)
  [flag_dvalid] -> Subsystem29/2(en)
  Subsystem29/1(current) -> pipeline176/1(d)
  Subsystem29/3(min) -> pipeline178/1(d)
  Subsystem29/2(max) -> pipeline177/1(d)
  [flag_time] -> Subsystem30/3(value)
  [cnt_rst] -> Subsystem30/1(rst)
  [flag_pktstart] -> Subsystem30/2(en)
  Subsystem30/1(current) -> pipeline179/1(d)
  Subsystem30/3(min) -> pipeline181/1(d)
  Subsystem30/2(max) -> pipeline180/1(d)
  pipeline170/1(q) -> flag_pktfreq_stats/1(out_current)
  pipeline171/1(q) -> flag_pktfreq_stats/2(out_max)
  pipeline172/1(q) -> flag_pktfreq_stats/3(out_min)
  pipeline175/1(q) -> flag_pktxindex_stats/3(out_min)
  pipeline174/1(q) -> flag_pktxindex_stats/2(out_max)
  pipeline173/1(q) -> flag_pktxindex_stats/1(out_current)
  pipeline176/1(q) -> flag_pktxoffset_stats/1(out_current)
  pipeline177/1(q) -> flag_pktxoffset_stats/2(out_max)
  pipeline178/1(q) -> flag_pktxoffset_stats/3(out_min)
  pipeline181/1(q) -> flag_time_stats/3(out_min)
  pipeline180/1(q) -> flag_time_stats/2(out_max)
  pipeline179/1(q) -> flag_time_stats/1(out_current)
  pipeline182/1(q) -> flag_epoch_lsw/1(out_reg)
  pipeline183/1(q) -> flag_epoch_msw/1(out_reg)
  pipeline184/1(q) -> sync_time_msw/1(out_reg)
  pipeline185/1(q) -> sync_time_lsw/1(out_reg)
  pipeline186/1(q) -> pack_in_dv_rate/1(out_dv_rate)
  pipeline187/1(q) -> pack_out_dv_rate/1(out_dv_rate)
  pipeline188/1(q) -> pack_dv_err/1(out_dvblock_err_cnt)
  Constant10/1 -> [ct_d256]
  Counter/1 -> [ct_pktfreq]
  Counter6/1 -> [ct_pkt_x_index]
  Counter9/1 -> [ct_pkt_x_offset]
  [sync80] -> time_gen/1(wr_sync_in)
  [valid80] -> time_gen/2(wr_en)
  [pfb_sync] -> time_gen/4(rd_sync_in)
  [pfb_dv] -> time_gen/5(rd_en)
  [pfb_d144_1] -> Concat1/2
  [pfb_d144_0] -> Concat1/1
  Concat1/1 -> time_gen/6(rd_misc_in)
  [time80] -> time_gen/3(wr_val_in)
  time_gen/1(rd_sync_out) -> [fdfs_sync]
  [ddc_sync] -> [pfb_sync]
  [ddc_dvalid] -> [pfb_dv]
  time_gen/2(rd_dvalid) -> [fdfs_dv]
  time_gen/4(rd_misc_out) -> Terminator/1
  Constant29/1 -> Concat2/2
  time_gen/3(rd_val_out) -> Concat2/1
  Concat2/1 -> [pfb_time]
  Convert/1 -> [pfb_d144_0]
  [ddc_pol0] -> Convert/1
  Convert4/1 -> [pfb_d144_1]
  [ddc_pol1] -> Convert4/1
